simulink model "WheelSpeeds"  (R2024b)
settings: Solver=FixedStepAuto  StartTime=0.0  StopTime=10.0  RelTol=1e-3
undefined symbols (not defined in the file): rGearboxRatio, rTyreRadius
settings Model: DataDictionary=Master_Dictionary.sldd  EnableAccessToBaseWorkspace=off  Creator=torni  LastModifiedBy=will
settings SolverCC: AlgebraicLoopSolver=TrustRegion
settings DataIOCC: ReturnWorkspaceOutputs=off
settings OptimizationCC: DefaultParameterBehavior=Inlined  EnhancedBackFolding=on  PassReuseOutputArgsAs=Individual arguments  ZeroExternalMemoryAtStartup=off  ZeroInternalMemoryAtStartup=off  OptimizeBlockOrder=speed  DifferentSizesBufferReuse=on  OptimizationCustomize=off  EfficientTunableParamExpr=on
settings DebuggingCC: ParameterTunabilityLossMsg=error  UnconnectedInputMsg=warning  UnconnectedOutputMsg=warning  UnconnectedLineMsg=warning  ArithmeticOperatorsInVariantConditions=warning
settings HardwareCC: TargetLargestAtomicInteger=Long  TargetLargestAtomicFloat=Double  TargetIntDivRoundTo=Zero  TargetEndianess=LittleEndian  TargetHWDeviceType=ARM Compatible->ARM Cortex-M  ProdEqTarget=off
settings ModelReferenceCC: EnableRefExpFcnMdlSchedulingChecks=on
settings SFSimCC: MATLABDynamicMemAlloc=off  CustomCodeUndefinedFunction=UseInterfaceOnly
settings RTWCC: Description=Embedded Coder  SystemTargetFile=ert.tlc  TemplateMakefile=ert_default_tmf  Toolchain=GNU Tools for ARM Embedded Processors  RTWCompilerOptimization=on  GPUComputeCapability=3.5
settings CodeAppCC: ForceParamTrailComments=on  IgnoreCustomStorageClasses=off  OperatorAnnotations=on  SimulinkDataObjDesc=on  SFDataObjDesc=on  InsertBlockDesc=on
settings ERTTargetCC: TargetLangStandard=C99 (ISO)  GenerateSampleERTMain=on  ERTCustomFileTemplate=example_file_process.tlc

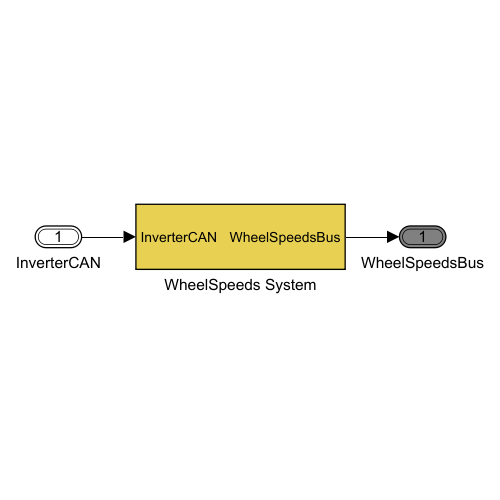
[thumbnail: Simulink's stored preview of the top-level diagram]
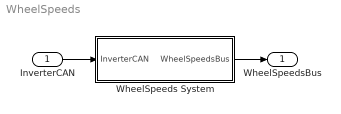
== system WheelSpeeds ==
  InverterCAN : Inport  OutDataTypeStr=Bus: CAN1_2Bus
  WheelSpeeds System : Subsystem
  WheelSpeedsBus : Outport  OutDataTypeStr=Bus: WheelSpeedsBus  VectorParamsAs1DForOutWhenUnconnected=off
  wires:
  InverterCAN/1 -> WheelSpeeds System/1(InverterCAN)
  WheelSpeeds System/1(WheelSpeedsBus) -> WheelSpeedsBus/1

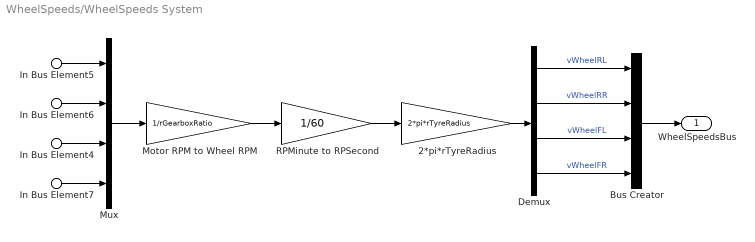
== system WheelSpeeds/WheelSpeeds System ==
  In Bus Element4 : Inport  PortName=InverterCAN  Element=InverterFLCANBus.nMotorFL
  In Bus Element5 : Inport  PortName=InverterCAN  Element=InverterRLCANBus.nMotorRL
  In Bus Element6 : Inport  PortName=InverterCAN  Element=InverterRRCANBus.nMotorRR
  In Bus Element7 : Inport  PortName=InverterCAN  Element=InverterFRCANBus.nMotorFR
  2*pi*rTyreRadius : Gain  Gain=2*pi*rTyreRadius
  Bus Creator : BusCreator  Inputs=4  OutDataTypeStr=Bus: WheelSpeedsBus
  Demux : Demux
  Motor RPM to Wheel RPM : Gain  Gain=1/rGearboxRatio
  Mux : Mux
  RPMinute to RPSecond : Gain  Gain=1/60
  WheelSpeedsBus : Outport  OutDataTypeStr=Bus: WheelSpeedsBus  VectorParamsAs1DForOutWhenUnconnected=off
  wires:
  Demux/1 -> Bus Creator/1  "vWheelRL"
  Demux/2 -> Bus Creator/2  "vWheelRR"
  Demux/4 -> Bus Creator/4  "vWheelFR"
  Demux/3 -> Bus Creator/3  "vWheelFL"
  In Bus Element5/1 -> Mux/1
  In Bus Element6/1 -> Mux/2
  In Bus Element4/1 -> Mux/3
  In Bus Element7/1 -> Mux/4
  RPMinute to RPSecond/1 -> 2*pi*rTyreRadius/1
  Mux/1 -> Motor RPM to Wheel RPM/1
  Motor RPM to Wheel RPM/1 -> RPMinute to RPSecond/1
  2*pi*rTyreRadius/1 -> Demux/1
  Bus Creator/1 -> WheelSpeedsBus/1
